simulink library "rfprivate1"  (Simulink 6.0)
settings: Solver=ode45  SolverMode=SingleTasking  StartTime=0.0  StopTime=10.0  RelTol=1e-3
undefined symbols (not defined in the file or in its folder): D, seed
libraries: rfprivate1 x6, dspsigattribs x4, dsparch4 x4, dspsrcs4 x1
settings Model: RequirementInfo=9  CovMetricSettings=d  Creator=tdelve  LastModifiedBy=mikem  ExtModeAutoUpdateStatusClock=off  ProdHWDeviceType=Specified
settings DataIOCC: SignalLoggingName=logsOut
settings OptimizationCC: BooleanDataType=off
settings DebuggingCC: CheckExecutionContextPreStartOutputMsg=on  CheckExecutionContextRuntimeOutputMsg=on  SolverPrmCheckMsg=none
settings HardwareCC: ProdHWDeviceType=Specified  TargetUnknown=on
settings ModelReferenceCC: UpdateModelReferenceTargets=IfOutOfDate
settings GRTTargetCC: LifeSpan=inf
settings SFSimCC: SFSimApplyToAllLibs=on  SFSimBuildMode=Incremental

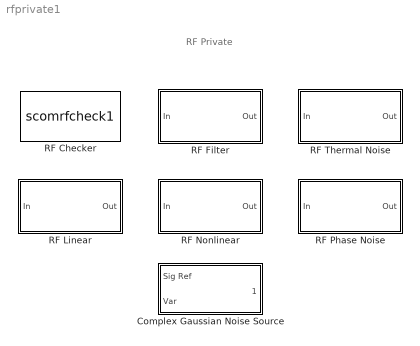
== system rfprivate1 ==
  note: RF Private
  Complex Gaussian Noise Source : Subsystem  EnableExecutionContextPropagation=on
  RF Checker : S-Function  FunctionName=scomrfcheck1  Parameters=ts  mask(RF Checker){ts=1e-6}
      mask prompts: ts "Sample time:"
      mask help: Check the input signal to RF physical blocks.
      mask Display: disp('RF Checker');
  RF Filter : Subsystem  EnableExecutionContextPropagation=on  mask(RF Filter){model=[], Ts=1e-6}
      mask prompts: model "Filter object:"; Ts "Sample time (s):"
      mask help:
      | This block performs complex baseband equivalent filtering based on complex impulse response that is calculated at RF frequencies.
      |
      | There is a delay through this block.
      mask init:
      | sresp = [];
      | if isa(model, 'rfmodel.filter')
      | 	sresp = get(model, 'ImpulseResp');
      | end
      | if isempty(sresp)
      | 	sresp = 1;
      | end
      mask Display: disp('RF Filter');
  RF Linear : Subsystem  EnableExecutionContextPropagation=on  mask(RF Linear){model=[]}
      mask prompts: model "Linear object:"
      mask help:
      | This block performs complex baseband equivalent filtering based on complex impulse response that is calculated from netwok parameters at RF frequencies.
      |
      | There is a delay through this block.
      mask init:
      | resp = [];
      | if isa(model, 'rfmodel.linear')
      | 	resp = get(model, 'ImpulseResp');
      | end
      | if isempty(resp)
      | 	resp = 1;
      | end
      mask Display: disp('RF Linear');
  RF Nonlinear : Subsystem  EnableExecutionContextPropagation=on  mask(RF Nonlinear){model=[]}
      mask prompts: model "Nonlinear object:"
      mask help: This block performs AMAM/AMPM nonlinear analysis.
      mask init:
      | method = 0;
      | if isa(model, 'rfmodel.nonlinear')
      | 	method = get(model, 'Method');
      | 	inputGain = get(model, 'InputEffect');
      | 	outputGain =  2.0/get(model, 'LinearGain');
      |     input = get(model, 'XData');
      | 	amam = get(model, 'AMAMData');
      |  	ampm = get(model, 'AMPMData');
      | end 
      | if method == 0
      | 	inputGain = 1;
      | 	outputGain = 1;
      |     input = [1:2];	
      |     amam = [1:2];	
      |     ampm = [1:2];
      | end
      mask Display: disp('RF Nonlinear');
  RF Phase Noise : Subsystem  EnableExecutionContextPropagation=on  mask(RF Phase Noise){model=[]}
      mask prompts: model "Nonlinear object:"
      mask help: Complex baseband model of RF phase noise.
      mask init:
      | resp = [];
      | if isa(model, 'rfmodel.nonlinear')
      | 	resp = get(model, 'PhaseNoiseResp');
      | 	seed = get(model, 'Seed');
      | 	method = 1;
      | end 
      | if isempty(resp)
      | 	resp = 1;
      |     seed = 0;
      | 	method = 0;
      | end
      settings: AttributesFormatString=\n
      mask Help: helpview(commbhelp)
      mask Display: disp('RF Phase Noise');
  RF Thermal Noise : Subsystem  EnableExecutionContextPropagation=on  mask(RF Thermal Noise){model=[]}
      mask prompts: model "System object:"
      mask help: This block performs complex baseband equivalent thermal noise.
      mask init:
      | resp = [];
      | if isa(model, 'rfmodel.system')
      | 	resp = get(model, 'NoiseResp');
      | 	seed = get(model, 'Seed');
      | end
      | if isempty(resp)
      |    resp = 0;
      |    seed = 67987111;
      | end
      mask Display: disp('RF Thermal Noise');

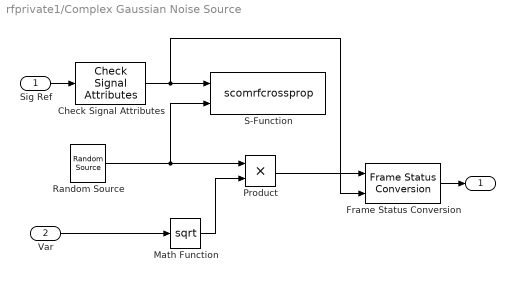
== system rfprivate1/Complex Gaussian Noise Source ==
  Sig Ref : Inport  LatchInput=off
  Var : Inport  Port=2  LatchInput=off
  Check Signal Attributes : dspsigattribs/Check Signal Attributes  SigAttribCheckMethod=Does not match attributes exactly  Complexity=Complex  Frame=Ignore  DimsCheckMethod=Ignore  Dimensions=1-D  DatatypeCheckMethod=Ignore  DatatypeGeneral=Boolean  DtypeFloatSpecific=Any floating-point  DtypeFixedSpecific=Any fixed-point  DtypeIntSpecific=Any integer  SampleMode=Ignore
  Frame Status Conversion : dspsigattribs/Frame Status Conversion  growRefPort=on  outframe=Frame-based
  Math Function : Math  Operator=sqrt  SaturateOnIntegerOverflow=on
  Product : Product  RndMeth=Zero
  Random Source : dspsrcs4/Random Source  SrcType=Gaussian  NormMethod=Ziggurat  CltLength=12  Min=0  Max=1  Mean=0  Var=1  RepMode=Specify seed  Seed=seed  Inherit=on  SampMode=Discrete  SampTime=1  SampFrame=1  DataType=Double  OutComplex=Real
  S-Function : S-Function  FunctionName=scomrfcrossprop
  " " : Outport
  wires:
  Sig Ref/1 -> Check Signal Attributes/1
  Random Source/1 -> Product/1, S-Function/2
  Var/1 -> Math Function/1
  Math Function/1 -> Product/2
  Product/1 -> Frame Status Conversion/1
  Frame Status Conversion/1 -> " "/1
  Check Signal Attributes/1 -> Frame Status Conversion/2, S-Function/1

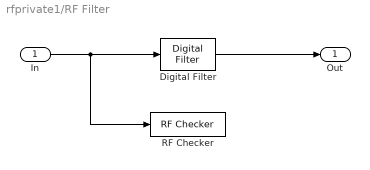
== system rfprivate1/RF Filter ==
  In : Inport  LatchInput=off
  Digital Filter : dsparch4/Digital Filter  TypePopup=FIR (all zeros)  IIRFiltStruct=Direct form II transposed  AllPoleFiltStruct=Direct form  FIRFiltStruct=Direct form  CoeffSource=Specify via dialog  NumCoeffs=sresp  DenCoeffs=1  BiQuadCoeffs=[1 0.3 0.4 1 0.1 0.2]  LatticeCoeffs=[0.2 0.4]  denIgnore=on  FiltPerSampPopup=One filter per frame  IC=0  ICnum=0  ICden=0  roundingMode=Floor  overflowMode=off
  RF Checker : rfprivate1/RF Checker  ts=Ts
  Out : Outport
  wires:
  Digital Filter/1 -> Out/1
  In/1 -> Digital Filter/1, RF Checker/1

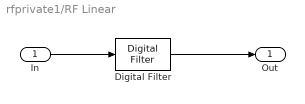
== system rfprivate1/RF Linear ==
  In : Inport  LatchInput=off
  Digital Filter : dsparch4/Digital Filter  TypePopup=FIR (all zeros)  IIRFiltStruct=Direct form II transposed  AllPoleFiltStruct=Direct form  FIRFiltStruct=Direct form  CoeffSource=Specify via dialog  NumCoeffs=resp  DenCoeffs=1  BiQuadCoeffs=[1 0.3 0.4 1 0.1 0.2]  LatticeCoeffs=[0.2 0.4]  denIgnore=on  FiltPerSampPopup=One filter per frame  IC=0  ICnum=0  ICden=0  roundingMode=Floor  overflowMode=off
  Out : Outport
  wires:
  In/1 -> Digital Filter/1
  Digital Filter/1 -> Out/1

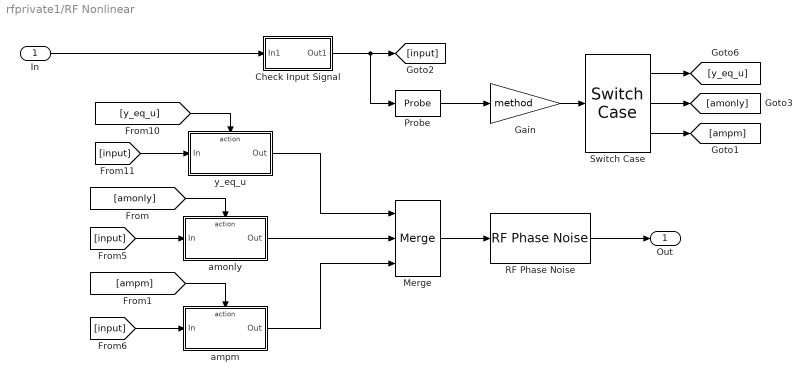
== system rfprivate1/RF Nonlinear ==
  In : Inport  LatchInput=off
  Check Input Signal : Subsystem  EnableExecutionContextPropagation=on
      mask Display: disp('Check\nInput Signal');
  Gain : Gain  Gain=method  SaturateOnIntegerOverflow=on
  Merge : Merge  Inputs=3
  Probe : Probe  ProbeWidth=off  ProbeSampleTime=off
  RF Phase Noise : rfprivate1/RF Phase Noise  model=model
      settings: AttributesFormatString=\n
  Switch Case : SwitchCase  CaseConditions={0 1 2}  CaseShowDefault=off
  amonly : Subsystem  TreatAsAtomicUnit=on  EnableExecutionContextPropagation=on
  ampm : Subsystem  TreatAsAtomicUnit=on  EnableExecutionContextPropagation=on
  y_eq_u : Subsystem  TreatAsAtomicUnit=on  EnableExecutionContextPropagation=on
  Out : Outport
  wires:
  Gain/1 -> Switch Case/1
  [amonly] -> amonly/Action
  [ampm] -> ampm/Action
  In/1 -> Check Input Signal/1(In1)
  Check Input Signal/1(Out1) -> [input], Probe/1
  [input] -> amonly/1(In)
  [input] -> ampm/1(In)
  Probe/1 -> Gain/1
  [y_eq_u] -> y_eq_u/Action
  [input] -> y_eq_u/1(In)
  ampm/1(Out) -> Merge/3
  amonly/1(Out) -> Merge/2
  y_eq_u/1(Out) -> Merge/1
  Switch Case/2 -> [amonly]
  Switch Case/3 -> [ampm]
  Switch Case/1 -> [y_eq_u]
  Merge/1 -> RF Phase Noise/1
  RF Phase Noise/1 -> Out/1

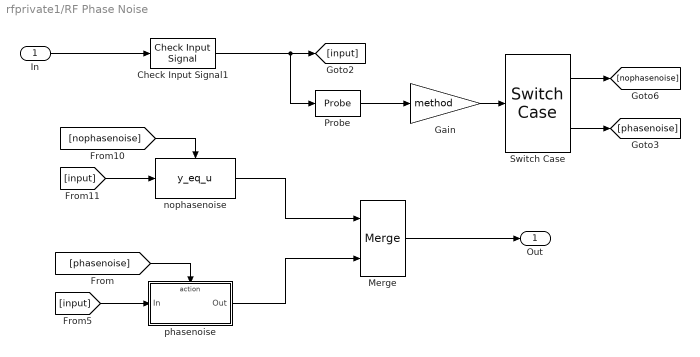
== system rfprivate1/RF Phase Noise ==
  In : Inport  LatchInput=off
  Check Input Signal1 : rfprivate1/RF Nonlinear/Check Input Signal
  Gain : Gain  Gain=method  SaturateOnIntegerOverflow=on
  Merge : Merge
  Probe : Probe  ProbeWidth=off  ProbeSampleTime=off
  Switch Case : SwitchCase  CaseConditions={0 1}  CaseShowDefault=off
  nophasenoise : rfprivate1/RF Nonlinear/y_eq_u
  phasenoise : Subsystem  AncestorBlock=rfprivate1/RF Nonlinear/amonly  TreatAsAtomicUnit=on  EnableExecutionContextPropagation=on
  Out : Outport
  wires:
  Gain/1 -> Switch Case/1
  [phasenoise] -> phasenoise/Action
  In/1 -> Check Input Signal1/1
  Check Input Signal1/1 -> [input], Probe/1
  Probe/1 -> Gain/1
  [nophasenoise] -> nophasenoise/Action
  [input] -> nophasenoise/1
  nophasenoise/1 -> Merge/1
  Switch Case/2 -> [phasenoise]
  Switch Case/1 -> [nophasenoise]
  Merge/1 -> Out/1
  [input] -> phasenoise/1(In)
  phasenoise/1(Out) -> Merge/2

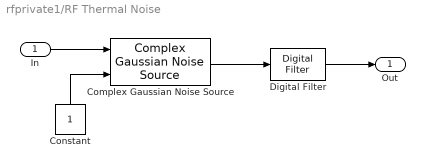
== system rfprivate1/RF Thermal Noise ==
  In : Inport  LatchInput=off
  Complex Gaussian Noise Source : rfprivate1/Complex Gaussian Noise Source
  Constant : Constant  Orientation=up  SampleTime=Inf
  Digital Filter : dsparch4/Digital Filter  TypePopup=FIR (all zeros)  IIRFiltStruct=Direct form II transposed  AllPoleFiltStruct=Direct form  FIRFiltStruct=Direct form  CoeffSource=Specify via dialog  NumCoeffs=resp  DenCoeffs=1  BiQuadCoeffs=[1 0.3 0.4 1 0.1 0.2]  LatticeCoeffs=[0.2 0.4]  denIgnore=on  FiltPerSampPopup=One filter per frame  IC=0  ICnum=0  ICden=0  roundingMode=Floor  overflowMode=off
  Out : Outport
  wires:
  In/1 -> Complex Gaussian Noise Source/1
  Complex Gaussian Noise Source/1 -> Digital Filter/1
  Digital Filter/1 -> Out/1
  Constant/1 -> Complex Gaussian Noise Source/2

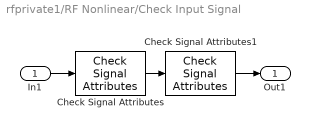
== system rfprivate1/RF Nonlinear/Check Input Signal ==
  In1 : Inport  LatchInput=off
  Check Signal Attributes : dspsigattribs/Check Signal Attributes  SigAttribCheckMethod=Does not match attributes exactly  Complexity=Complex  Frame=Ignore  DimsCheckMethod=Is...  Dimensions=Column vector (2-D) or scalar  DatatypeCheckMethod=Ignore  DatatypeGeneral=Boolean  DtypeFloatSpecific=Any floating-point  DtypeFixedSpecific=Any fixed-point  DtypeIntSpecific=Any integer  SampleMode=Ignore
  Check Signal Attributes1 : dspsigattribs/Check Signal Attributes  SigAttribCheckMethod=Matches attributes exactly  Complexity=Ignore  Frame=Sample-based  DimsCheckMethod=Is...  Dimensions=Vector (1-D or 2-D)  DatatypeCheckMethod=Ignore  DatatypeGeneral=Boolean  DtypeFloatSpecific=Any floating-point  DtypeFixedSpecific=Any fixed-point  DtypeIntSpecific=Any integer  SampleMode=Ignore
  Out1 : Outport
  wires:
  Check Signal Attributes/1 -> Check Signal Attributes1/1
  Check Signal Attributes1/1 -> Out1/1
  In1/1 -> Check Signal Attributes/1

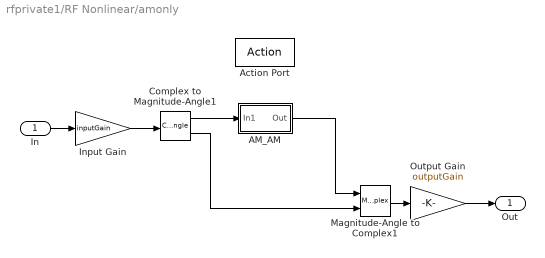
== system rfprivate1/RF Nonlinear/amonly ==
  In : Inport  LatchInput=off
  Action Port : ActionPort
  AM_AM : Subsystem  EnableExecutionContextPropagation=on
      mask Display: disp('AM/AM')
  Complex to Magnitude-Angle1 : ComplexToMagnitudeAngle
  Input Gain : Gain  Gain=inputGain  SaturateOnIntegerOverflow=on
  Magnitude-Angle to Complex1 : MagnitudeAngleToComplex
  Output Gain : Gain  Gain=outputGain  SaturateOnIntegerOverflow=on
  Out : Outport
  wires:
  Output Gain/1 -> Out/1
  In/1 -> Input Gain/1
  Input Gain/1 -> Complex to Magnitude-Angle1/1
  Magnitude-Angle to Complex1/1 -> Output Gain/1
  AM_AM/1(Out) -> Magnitude-Angle to Complex1/1
  Complex to Magnitude-Angle1/1 -> AM_AM/1(In1)
  Complex to Magnitude-Angle1/2 -> Magnitude-Angle to Complex1/2

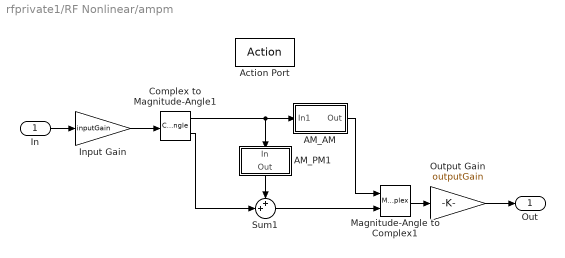
== system rfprivate1/RF Nonlinear/ampm ==
  In : Inport  LatchInput=off
  Action Port : ActionPort
  AM_AM : Subsystem  EnableExecutionContextPropagation=on
      mask Display: disp('AM/AM')
  AM_PM1 : Subsystem  Orientation=down  EnableExecutionContextPropagation=on
      mask Display: disp('AM/PM')
  Complex to Magnitude-Angle1 : ComplexToMagnitudeAngle
  Input Gain : Gain  Gain=inputGain  SaturateOnIntegerOverflow=on
  Magnitude-Angle to Complex1 : MagnitudeAngleToComplex
  Output Gain : Gain  Gain=outputGain  SaturateOnIntegerOverflow=on
  Sum1 : Sum  Inputs=++|  SaturateOnIntegerOverflow=on  InputSameDT=on
  Out : Outport
  wires:
  Complex to Magnitude-Angle1/1 -> AM_PM1/1(In), AM_AM/1(In1)
  AM_AM/1(Out) -> Magnitude-Angle to Complex1/1
  Magnitude-Angle to Complex1/1 -> Output Gain/1
  Input Gain/1 -> Complex to Magnitude-Angle1/1
  Complex to Magnitude-Angle1/2 -> Sum1/2
  In/1 -> Input Gain/1
  Output Gain/1 -> Out/1
  AM_PM1/1(Out) -> Sum1/1
  Sum1/1 -> Magnitude-Angle to Complex1/2

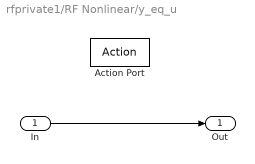
== system rfprivate1/RF Nonlinear/y_eq_u ==
  In : Inport  LatchInput=off
  Action Port : ActionPort
  Out : Outport
  wires:
  In/1 -> Out/1

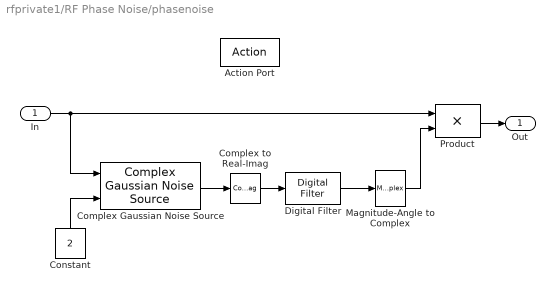
== system rfprivate1/RF Phase Noise/phasenoise ==
  In : Inport  LatchInput=off
  Action Port : ActionPort
  Complex Gaussian Noise Source : rfprivate1/Complex Gaussian Noise Source
  Complex to Real-Imag : ComplexToRealImag  Output=Real
  Constant : Constant  Orientation=up  Value=2  SampleTime=Inf
  Digital Filter : dsparch4/Digital Filter  TypePopup=FIR (all zeros)  IIRFiltStruct=Direct form II transposed  AllPoleFiltStruct=Direct form  FIRFiltStruct=Direct form  CoeffSource=Specify via dialog  NumCoeffs=resp  DenCoeffs=1  BiQuadCoeffs=[1 0.3 0.4 1 0.1 0.2]  LatticeCoeffs=[0.2 0.4]  denIgnore=on  FiltPerSampPopup=One filter per frame  IC=0  ICnum=0  ICden=0  roundingMode=Floor  overflowMode=off
  Magnitude-Angle to Complex : MagnitudeAngleToComplex  Input=Angle  ConstantPart=1
  Product : Product  SaturateOnIntegerOverflow=on  InputSameDT=on
  Out : Outport
  wires:
  Digital Filter/1 -> Magnitude-Angle to Complex/1
  Magnitude-Angle to Complex/1 -> Product/2
  In/1 -> Product/1, Complex Gaussian Noise Source/1
  Product/1 -> Out/1
  Complex to Real-Imag/1 -> Digital Filter/1
  Constant/1 -> Complex Gaussian Noise Source/2
  Complex Gaussian Noise Source/1 -> Complex to Real-Imag/1

== system rfprivate1/RF Nonlinear/amonly/AM_AM ==
  In1 : Inport  LatchInput=off
  Look-Up Table : Lookup  DialogController=Simulink.DDGSource  InputValues=input  OutputValues=amam  LookUpMeth=Interpolation-Use End Values
  Out : Outport
  wires:
  In1/1 -> Look-Up Table/1
  Look-Up Table/1 -> Out/1

== system rfprivate1/RF Nonlinear/ampm/AM_AM ==
  In1 : Inport  LatchInput=off
  Look-Up Table : Lookup  DialogController=Simulink.DDGSource  InputValues=input  OutputValues=amam  LookUpMeth=Interpolation-Use End Values
  Out : Outport
  wires:
  Look-Up Table/1 -> Out/1
  In1/1 -> Look-Up Table/1

== system rfprivate1/RF Nonlinear/ampm/AM_PM1 ==
  In : Inport  LatchInput=off
  Look-Up Table : Lookup  DialogController=Simulink.DDGSource  InputValues=input  OutputValues=ampm
  Out : Outport
  wires:
  Look-Up Table/1 -> Out/1
  In/1 -> Look-Up Table/1
